simulink model "flanger"  (R2019a)
settings: Solver=VariableStepAuto  StartTime=0.0  StopTime=30  RelTol=1e-3
libraries: dspvision x1, dspsrcs4 x1, dspobslib x1, Librairie x1, dspsigops x1
settings Model: Creator=Ahmed  LastModifiedBy=Ahmed

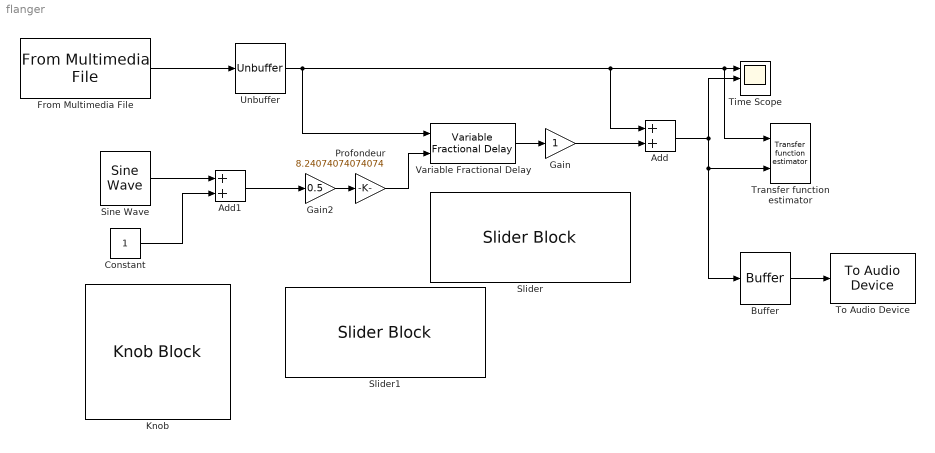
== system flanger ==
  Add : Sum
  Add1 : Sum
  Buffer : Buffer  N=1024  OutputFrames=off
  Constant : Constant
  From Multimedia File : dspvision/From Multimedia File  inputFilename=C:\Users\Ahmed\Nextcloud\L3\LU3EE105\Audio\Documents de TP et projet-20191118\Projet\because.wav  readRange=[1 Inf]  loop=on  numPlays=inf  outputStreams=Audio only  videoDataType=single  audioDataType=double  inheritSampleTime=on  userDefinedSampleTime=1/30  noAudioOutput=off  isIntensityVideo=off  fourcc=RGB  colorVideoFormat=Separate color signals  outputEOF=off  dataOrg=Column-major  audioFrameSize=1024  computeAudioFrameSize=off  outSamplingMode=Sample based
      settings: SourceProductName=DSP System Toolbox  SourceProductBaseCode=DS
  Gain : Gain
  Gain2 : Gain  Gain=0.5
  Knob : KnobBlock  ScaleMax=20
  Profondeur : Gain  Gain=8.24074074074074
  Sine Wave : dspsrcs4/Sine Wave  Amplitude=1  Frequency=1.620863596598307  Phase=0  SampleMode=Discrete  OutComplex=Real  CompMethod=Trigonometric fcn  TableSize=Speed  SampleTime=1/48000  SamplesPerFrame=1  ResetState=Restart at time zero  OutputFrames=off  dataType=double  wordLen=16  udDataType=sfix(16)  fracBitsMode=Best precision  numFracBits=15  OutDataTypeStr=double  LastOutDataTypeStr=double
  Slider : SliderBlock  ScaleMax=1
  Slider1 : SliderBlock  ScaleMax=10
  Time Scope : Scope  NumInputPorts=3
  To Audio Device : dspobslib/To Audio Device  deviceName=Default  inheritSampleRate=on  sampleRate=44100  deviceDatatype=Determine from input data type  autoBufferSize=on  bufferSize=4096  queueDuration=1.0  defaultOutputChannelMapping=on  outputChannelMapping=1:2  outputNumUnderrunSamples=off
      settings: SourceProductName=DSP System Toolbox  SourceProductBaseCode=DS
  Transfer function estimator : Librairie/Transfer function estimator  fee=11025  NN=1024
  Unbuffer : Unbuffer
  Variable Fractional Delay : dspsigops/Variable Fractional Delay  mode=OBSOLETE  modeActive=Linear  L=4  FarrowL=4  R=10  alpha=1  dmax=100  InputProcessing=Columns as channels (frame based)  ic=0  noDFT=off  fallbackFIR=Clip to the minimum value necessary for centered kernel  fallbackFarrow=Clip to the minimum value necessary for centered kernel  roundingMode=Zero  overflowMode=off
      settings: SourceProductName=DSP System Toolbox  SourceProductBaseCode=DS
  wires:
  Constant/1 -> Add1/2
  Variable Fractional Delay/1 -> Gain/1
  From Multimedia File/1 -> Unbuffer/1
  Add/1 -> Transfer function estimator/2, Buffer/1, Time Scope/2
  Gain/1 -> Add/2
  Buffer/1 -> To Audio Device/1
  Add1/1 -> Gain2/1
  Sine Wave/1 -> Add1/1
  Unbuffer/1 -> Variable Fractional Delay/1, Transfer function estimator/1, Time Scope/1, Add/1
  Profondeur/1 -> Variable Fractional Delay/2
  Gain2/1 -> Profondeur/1
